simulink model "test3"  (Simulink 7.4)
settings: Solver=ode45  StartTime=0.0  StopTime=10.0  RelTol=1e-3
libraries: Copter_Library x1
settings Model: Creator=alstit04  LastModifiedBy=alstit04

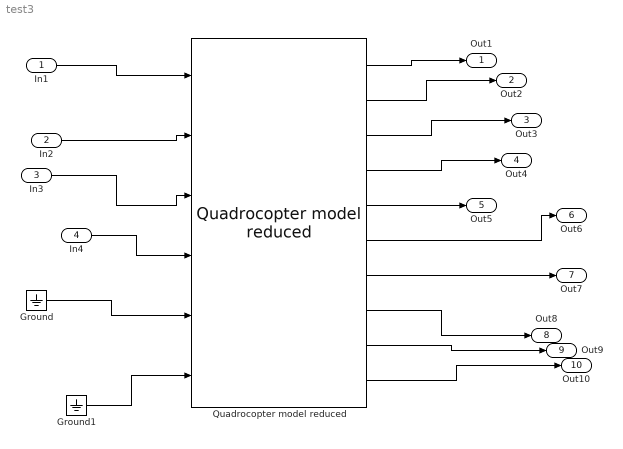
== system test3 ==
  In1 : Inport  OutDataType=fixdt(1, 16)  OutScaling=2^0
  In2 : Inport  Port=2  OutDataType=fixdt(1, 16)  OutScaling=2^0
  In3 : Inport  Port=3  OutDataType=fixdt(1, 16)  OutScaling=2^0
  In4 : Inport  Port=4  OutDataType=fixdt(1, 16)  OutScaling=2^0
  Ground : Ground
  Ground1 : Ground
  Quadrocopter model reduced : Copter_Library/Quadrocopter model reduced  SystemSampleTime=-1
  Out1 : Outport  OutDataType=fixdt(1, 16)  OutScaling=2^0
  Out2 : Outport  Port=2  OutDataType=fixdt(1, 16)  OutScaling=2^0
  Out3 : Outport  Port=3  OutDataType=fixdt(1, 16)  OutScaling=2^0
  Out4 : Outport  Port=4  OutDataType=fixdt(1, 16)  OutScaling=2^0
  Out5 : Outport  Port=5  OutDataType=fixdt(1, 16)  OutScaling=2^0
  Out6 : Outport  Port=6  OutDataType=fixdt(1, 16)  OutScaling=2^0
  Out7 : Outport  Port=7  OutDataType=fixdt(1, 16)  OutScaling=2^0
  Out8 : Outport  Port=8  OutDataType=fixdt(1, 16)  OutScaling=2^0
  Out9 : Outport  Port=9  OutDataType=fixdt(1, 16)  OutScaling=2^0
  Out10 : Outport  Port=10  OutDataType=fixdt(1, 16)  OutScaling=2^0
  wires:
  In3/1 -> Quadrocopter model reduced/3
  In2/1 -> Quadrocopter model reduced/2
  In1/1 -> Quadrocopter model reduced/1
  In4/1 -> Quadrocopter model reduced/4
  Ground/1 -> Quadrocopter model reduced/5
  Ground1/1 -> Quadrocopter model reduced/6
  Quadrocopter model reduced/1 -> Out1/1
  Quadrocopter model reduced/2 -> Out2/1
  Quadrocopter model reduced/3 -> Out3/1
  Quadrocopter model reduced/4 -> Out4/1
  Quadrocopter model reduced/5 -> Out5/1
  Quadrocopter model reduced/6 -> Out6/1
  Quadrocopter model reduced/7 -> Out7/1
  Quadrocopter model reduced/8 -> Out8/1
  Quadrocopter model reduced/9 -> Out9/1
  Quadrocopter model reduced/10 -> Out10/1
